simulink model "logic_controller"  (R2025b)
settings: Solver=VariableStepAuto  StartTime=0.0  StopTime=50  RelTol=1e-3
settings Model: Creator=alexandercushen  LastModifiedBy=alexandercushen

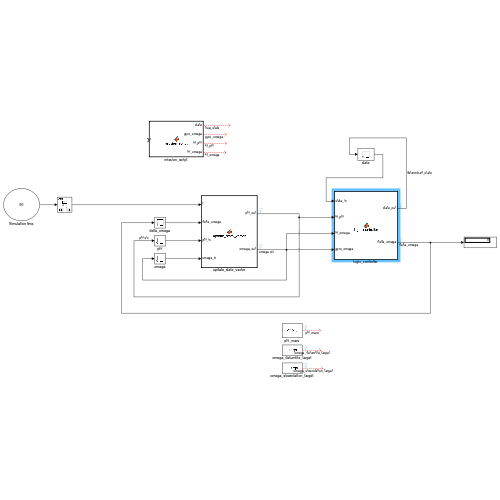
[thumbnail: Simulink's stored preview of the top-level diagram]
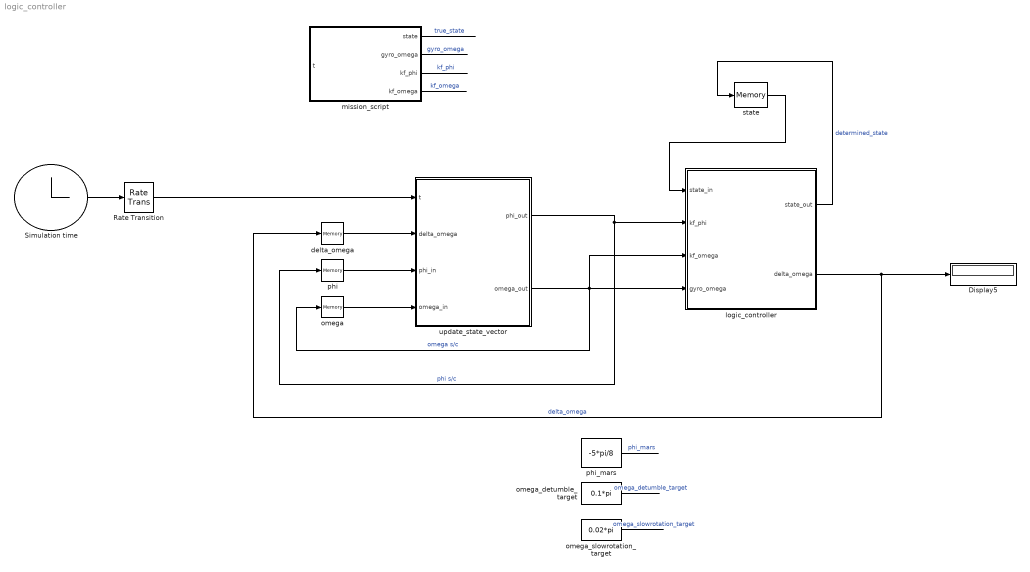
== system logic_controller ==
  Display5 : Display
  Rate Transition : RateTransition  OutPortSampleTime=0.025
  Simulation time : Clock
      settings: Decimation=2
  delta_omega : Memory
  logic_controller : MATLAB Function  TreatAsAtomicUnit=on
  mission_script : MATLAB Function  TreatAsAtomicUnit=on
  omega : Memory  InitialCondition=6
  omega_detumble_target : Constant  Value=0.1*pi
  omega_slowrotation_target : Constant  Value=0.02*pi
  phi : Memory  InitialCondition=1
  phi_mars : Constant  Value=-5*pi/8
  state : Memory
  update_state_vector : MATLAB Function  TreatAsAtomicUnit=on
  wires:
  Simulation time/1 -> Rate Transition/1
  logic_controller/1(state_out) -> state/1  "determined_state"
  state/1 -> logic_controller/1(state_in)
  Rate Transition/1 -> update_state_vector/1(t)
  update_state_vector/1(phi_out) -> phi/1, logic_controller/2(kf_phi)  "phi s/c"
  mission_script/1(state) -> ?  "true_state"
  mission_script/2(gyro_omega) -> ?  "gyro_omega"
  mission_script/3(kf_phi) -> ?  "kf_phi"
  mission_script/4(kf_omega) -> ?  "kf_omega"
  update_state_vector/2(omega_out) -> logic_controller/3(kf_omega), logic_controller/4(gyro_omega), omega/1  "omega s/c"
  phi/1 -> update_state_vector/3(phi_in)
  omega/1 -> update_state_vector/4(omega_in)
  logic_controller/2(delta_omega) -> delta_omega/1, Display5/1  "delta_omega"
  delta_omega/1 -> update_state_vector/2(delta_omega)
  phi_mars/1 -> ?  "phi_mars"
  omega_detumble_target/1 -> ?  "omega_detumble_target"
  omega_slowrotation_target/1 -> ?  "omega_slowrotation_target"

== matlab function logic_controller/logic_controller ==
  data: state_in input; kf_phi input; kf_omega input; gyro_omega input; state_out output; delta_omega output
function [state_out,delta_omega] = logic_controller(state_in,kf_phi,kf_omega,gyro_omega)

    % State controller parameters
    omega_detumble_target = 0.1*pi; % Target slew rate for detumble phase
    phi_starfield_min = -3*pi/4; % S/C attitude minimum to see star field
    phi_starfield_max = -pi/4; % S/C attitude maximum to see star field
    omega_slowrotation_target = 0.02*pi; % Target slew rate for slowrotation phase
    phi_mars = -5*pi/8; % Position of mars
    phi_mars_delta = pi/32; % Field of view tolerance for imaging mars
    omega_imaging_target = omega_slowrotation_target; % Maximum slew rate allowable for science imaging

    % By default, assume state_out = state_in and no actions are to be
    % taken
    state_out = state_in;
    delta_omega = 0;

    % S0: Detubmble
    if state_in == 0
        
        % Read gyro output directly
        omega = gyro_omega;
        
        % Check if we have achieved the goal for this state: sufficiently
        % slow rotation
        if abs(omega) < omega_detumble_target

            state_out = 1;
        
        % If not, proceed    
        else

            % Set delta_omega to try and null out spin
            delta_omega = -omega;


        end
    
    
    
    % S1: Slow rotation / coarse pointing
    elseif state_in == 1

        % Read from kalman filter
        phi = kf_phi;
        omega = kf_omega;

        % Check if we have achieved the goal for this state: very slow rotation, and
        % visibility of the star field
        omega_requirement = abs(omega) < omega_slowrotation_target;
        phi_requirement = phi > phi_starfield_min && phi < phi_starfield_max;

        % If so, move to next state
        if omega_requirement && phi_requirement

            state_out = 2;

        % If not, proceed with this state
        else
            
            % Check if we need to move back to S0
            if abs(omega) > omega_detumble_target 

                state_out = 0;
        
            % We are either spinning too fast, or not within the right
            % attitude range. First, if we are within the attitude range,
            % try to null out spin
            elseif phi_requirement

                delta_omega = -kf_omega;
            
            % If we are not within the
            % desired attitude range, then try to spin in the direction we
            % are already going at 2x omega_slowrotation_target
            else
                
                if omega>0

                    delta_omega = 2*omega_slowrotation_target - omega;

                else

                    delta_omega = - (2*omega_slowrotation_target - abs(omega));
                
                end

            end

        end

    % S3: Fine Pointing
    elseif state_in == 2
    
        % Read from kalman filter
        phi = kf_phi;
        omega = kf_omega;

        % Check if we have achieved the goal for this state: pointing at
        % Mars within FOV bounds, with slow enough rotation for imaging
        phi_requirement = phi > phi_mars-phi_mars_delta && phi < phi_mars + phi_mars_delta;
        omega_requirement = abs(omega) < omega_imaging_target;
        
        % If so, move to next state
        if phi_requirement && omega_requirement
            
            state_out = 3;

        % If not, proceed with this state
        else

            % First, check if we need to bump back up to S1, if we have
            % started spinning too fast or left the starfield
            if phi < phi_starfield_min || phi > phi_starfield_max || abs(omega) > 5*omega_slowrotation_target

                state_out = 1;
            
            % Getting to this stage means we are viewing the starfield,
            % spinning relatively slowly. Therefore, slew towards Mars

            % Our slew rate will depend on how far we are from the desired
            % attitude window.
            elseif phi-phi_mars > 5*phi_mars_delta

                delta_omega =  - (omega_slowrotation_target + omega);

            elseif phi-phi_mars < 5*phi_mars_delta

                delta_omega = (omega_slowrotation_target + omega);

             elseif phi-phi_mars > 2*phi_mars_delta

                delta_omega =  - (omega_slowrotation_target/2 + omega);

            elseif phi-phi_mars < 2*phi_mars_delta

                delta_omega = (omega_slowrotation_target/2 + omega);

           % Finally, if we are within the attitude range, null out
           % velocity
            elseif abs(phi-phi_mars) < phi_mars_delta

                delta_omega = -omega;

            end
                
    end
    
end

== matlab function logic_controller/mission_script ==
  data: state output; t input; gyro_omega output; kf_phi output; kf_omega output
function [state,gyro_omega,kf_phi,kf_omega] = mission_script(t)
    
    script_num = 1;

    mars_phi = -pi/2;
    
    % First mission simulation: nominal
    if script_num == 1
        
        % Script free parameters
        omega_0 = 2*pi; % Initial spin [rad/sec]
        omega_1 = 0.1*pi; % Spin rate after detumble [rad/sec] 
        phi_1 = -3*pi/4; % Attitude after despin, start of slow rotation [rad]
        phi_2 = -pi/4; % Attitude at start of fine point
        spindown_time = 10; % [s]
        finepoint_time = 20; % [s]
        wait_time = 2; % [s]
        omega_noise = 0.005*pi;
        phi_noise = 0.02;
  
        slowrotation_time = (phi_2-phi_1)/omega_1;

        % S0: detumble
        if t<spindown_time

            gyro_omega = omega_0 - (omega_0-omega_1)/spindown_time * t;
            kf_phi = nan;
            kf_omega = nan;
        
            state = 0;

        % S1: Slow Rotation
        elseif t<spindown_time+slowrotation_time
            
            gyro_omega = omega_1;
            kf_omega = omega_1;
            kf_phi = phi_1 + omega_1*(t-spindown_time);

            state = 1;

         % S2: Fine point
        elseif t<spindown_time+slowrotation_time+finepoint_time

            epoch_time = t-(spindown_time+slowrotation_time);

            if epoch_time < wait_time
                gyro_omega = 0;
                kf_phi = phi_2;
                kf_omega = 0;

            elseif epoch_time < finepoint_time - wait_time
                
                gyro_omega = (mars_phi - phi_2) / (finepoint_time - 2*wait_time);
                kf_phi = phi_2 + gyro_omega * (epoch_time-wait_time);
                kf_omega = gyro_omega;

            else

                gyro_omega = 0;
                kf_phi = mars_phi;
                kf_omega = 0;

            end

            state = 2;
            
        % S3: Science operation
        elseif t < spindown_time+slowrotation_time+finepoint_time+wait_time

            gyro_omega = 0;
            kf_phi = mars_phi;
            kf_omega = 0;

            state = 3;

        % S4: R.W. desaturation
        else

            gyro_omega = 0;
            kf_phi = mars_phi;
            kf_omega = 0;

            state = 4;
            
        end
    
    gyro_omega = gyro_omega + randn()*omega_noise;
    kf_phi = kf_phi + randn()*phi_noise;
    kf_omega = kf_omega + randn()*omega_noise/2;
    end
   
end

== matlab function logic_controller/update_state_vector ==
  data: t input; delta_omega input; phi_in input; phi_out output; omega_in input; omega_out output
function [phi_out,omega_out] = update_state_vector(t, delta_omega, phi_in, omega_in)

    dt = 0.025;
    phi_noise = 0.005;
    omega_noise = 0.01;
    magnetorquer_pulse = 0.05;
    magnetorquer_noise = 0.01;

    if delta_omega > 0

        omega_impulse = magnetorquer_pulse + randn()*magnetorquer_noise;

    elseif delta_omega < 0

        omega_impulse = -magnetorquer_pulse + randn()*magnetorquer_noise;

    else

        omega_impulse = 0;

    end

    omega_out = omega_in + randn()*omega_noise + omega_impulse;

    phi_out = wrapToPi(phi_in + dt*omega_in + randn()*phi_noise);


end
